simulink model "SCAUN_NOBIL"  (R2020a)
settings: Solver=VariableStepAuto  StartTime=0.0  StopTime=35  RelTol=1e-3
model workspace: external: MATLAB File E:\LICENTA\V6.0 - Model nou rotit Iunie\SCAUN_NOBIL_DataFile1.m (data not in the file)
undefined symbols (not defined in the file or in its folder): magnitude, sigbuilder_block, smiData, X, Y, Z
libraries: sm_lib x88, nesl_utility x19, simulink_extras x1
(part 1 of 3)
settings Model: Creator=Sebastian  LastModifiedBy=Sebastian

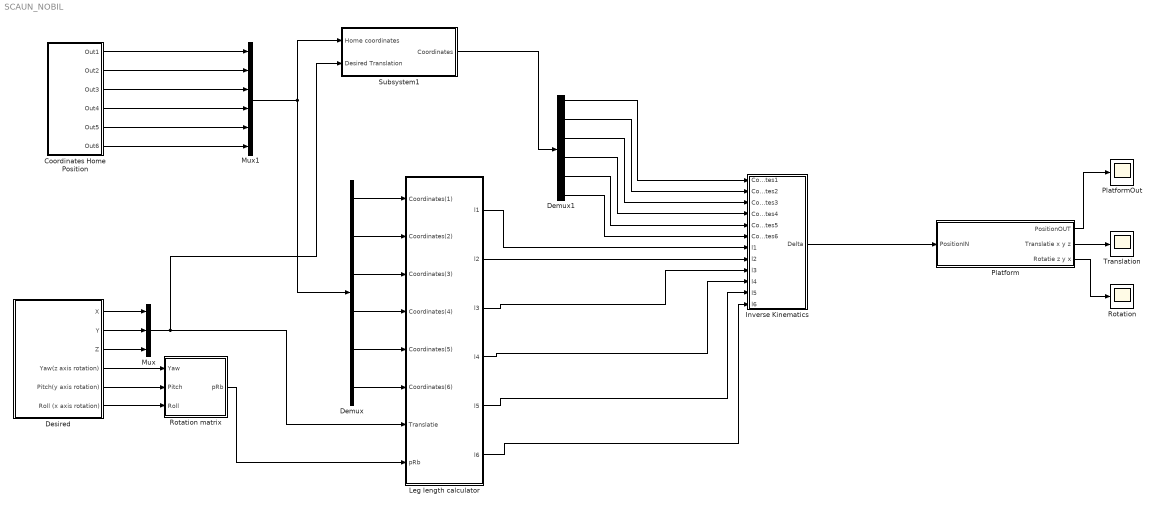
== system SCAUN_NOBIL ==
  Coordinates Home Position : Subsystem  TreatAsAtomicUnit=on
  Demux : Demux  Outputs=6
  Demux1 : Demux  Outputs=6
  Desired : Subsystem
  Inverse Kinematics : Subsystem
  Leg length calculator : Subsystem
  Mux : Mux  Inputs=3
  Mux1 : Mux  Inputs=6
  Platform : Subsystem
  PlatformOut : Scope
  Rotation : Scope
  Rotation matrix : Subsystem
  Subsystem1 : Subsystem
  Translation : Scope
  wires:
  Leg length calculator/6(l6) -> Inverse Kinematics/12(l6)
  Rotation matrix/1(pRb) -> Leg length calculator/8(pRb)
  Desired/2(Y) -> Mux/2
  Subsystem1/1(Coordinates) -> Demux1/1
  Inverse Kinematics/1(Delta) -> Platform/1(PositionIN)
  Platform/1(PositionOUT) -> PlatformOut/1
  Leg length calculator/5(l5) -> Inverse Kinematics/11(l5)
  Leg length calculator/4(l4) -> Inverse Kinematics/10(l4)
  Leg length calculator/3(l3) -> Inverse Kinematics/9(l3)
  Mux1/1 -> Demux/1, Subsystem1/1(Home coordinates)
  Desired/5(Pitch(y axis rotation)) -> Rotation matrix/2(Pitch)
  Coordinates Home Position/3(Out3) -> Mux1/3
  Coordinates Home Position/2(Out2) -> Mux1/2
  Demux1/4 -> Inverse Kinematics/4(Coordinates4)
  Platform/3(Rotatie z y x) -> Rotation/1
  Mux/1 -> Subsystem1/2(Desired Translation), Leg length calculator/7(Translatie)
  Desired/6(Roll (x axis rotation)) -> Rotation matrix/3(Roll)
  Leg length calculator/2(l2) -> Inverse Kinematics/8(l2)
  Coordinates Home Position/5(Out5) -> Mux1/5
  Leg length calculator/1(l1) -> Inverse Kinematics/7(l1)
  Demux/3 -> Leg length calculator/3(Coordinates(3))
  Demux1/5 -> Inverse Kinematics/5(Coordinates5)
  Coordinates Home Position/4(Out4) -> Mux1/4
  Demux/1 -> Leg length calculator/1(Coordinates(1))
  Demux1/1 -> Inverse Kinematics/1(Coordinates1)
  Coordinates Home Position/1(Out1) -> Mux1/1
  Platform/2(Translatie x y z) -> Translation/1
  Demux/5 -> Leg length calculator/5(Coordinates(5))
  Demux/6 -> Leg length calculator/6(Coordinates(6))
  Demux/2 -> Leg length calculator/2(Coordinates(2))
  Demux1/6 -> Inverse Kinematics/6(Coordinates6)
  Desired/1(X) -> Mux/1
  Demux1/2 -> Inverse Kinematics/2(Coordinates2)
  Demux1/3 -> Inverse Kinematics/3(Coordinates3)
  Desired/4(Yaw(z axis rotation)) -> Rotation matrix/1(Yaw)
  Demux/4 -> Leg length calculator/4(Coordinates(4))
  Desired/3(Z) -> Mux/3
  Coordinates Home Position/6(Out6) -> Mux1/6

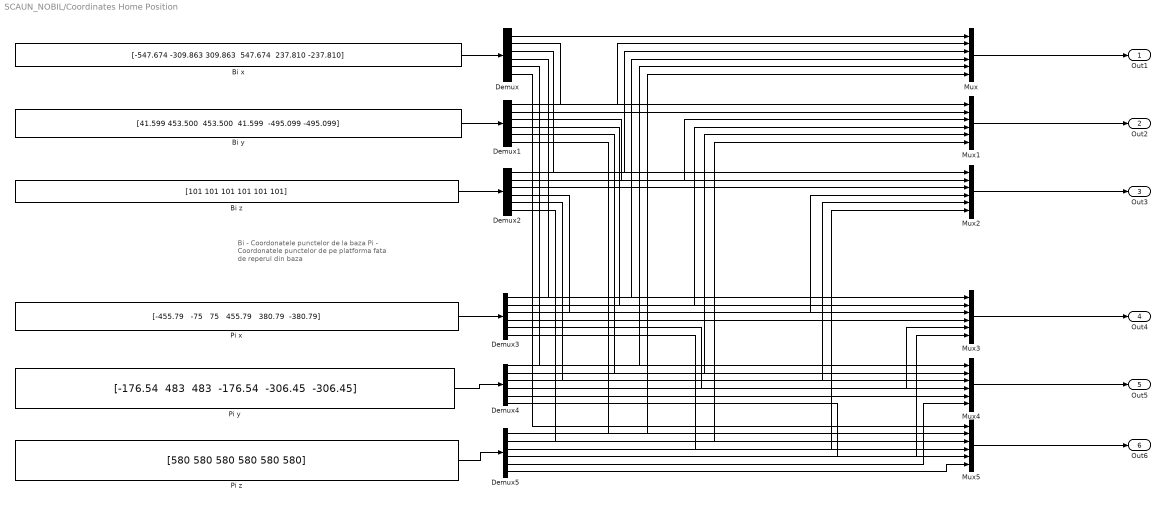
== system SCAUN_NOBIL/Coordinates Home Position ==
  note: Bi - Coordonatele punctelor de la baza
      | Pi - Coordonatele punctelor de pe platforma
      |       fata de reperul din baza
  Bi x : Constant  Value="[-547.674 -309.863 309.863  547.674  237.810 -237.810]"
  Bi y : Constant  Value="[41.599 453.500  453.500  41.599  -495.099 -495.099]"
  Bi z : Constant  Value=[101 101 101 101 101 101]
  Demux{,1..5} (6 alike) : Demux  Outputs=6
  Mux{,1..5} (6 alike) : Mux  Inputs=6
  Pi x : Constant  Value="[-455.79   -75   75   455.79   380.79  -380.79]"
  Pi y : Constant  Value="[-176.54  483  483  -176.54  -306.45  -306.45]"
  Pi z : Constant  Value=[580 580 580 580 580 580]
  Out1 : Outport
  Out2 : Outport  Port=2
  Out3 : Outport  Port=3
  Out4 : Outport  Port=4
  Out5 : Outport  Port=5
  Out6 : Outport  Port=6
  wires:
  Bi x/1 -> Demux/1
  Bi y/1 -> Demux1/1
  Bi z/1 -> Demux2/1
  Pi x/1 -> Demux3/1
  Pi y/1 -> Demux4/1
  Pi z/1 -> Demux5/1
  Demux/1 -> Mux/1
  Demux/2 -> Mux1/1
  Demux/3 -> Mux2/1
  Demux/4 -> Mux3/1
  Demux/5 -> Mux4/1
  Demux/6 -> Mux5/1
  Demux1/1 -> Mux/2
  Demux1/2 -> Mux1/2
  Demux1/3 -> Mux2/2
  Demux1/4 -> Mux3/2
  Demux1/5 -> Mux4/2
  Demux1/6 -> Mux5/2
  Demux2/1 -> Mux/3
  Demux2/2 -> Mux1/3
  Demux2/3 -> Mux2/3
  Demux2/4 -> Mux3/3
  Demux2/5 -> Mux4/3
  Demux2/6 -> Mux5/3
  Demux3/1 -> Mux/4
  Demux3/2 -> Mux1/4
  Demux3/3 -> Mux2/4
  Demux3/4 -> Mux3/4
  Demux3/5 -> Mux4/4
  Demux3/6 -> Mux5/4
  Demux4/1 -> Mux/5
  Demux4/2 -> Mux1/5
  Demux4/3 -> Mux2/5
  Demux4/4 -> Mux3/5
  Demux4/5 -> Mux4/5
  Demux4/6 -> Mux5/5
  Demux5/1 -> Mux/6
  Demux5/2 -> Mux1/6
  Demux5/3 -> Mux2/6
  Demux5/4 -> Mux3/6
  Demux5/5 -> Mux4/6
  Demux5/6 -> Mux5/6
  Mux/1 -> Out1/1
  Mux1/1 -> Out2/1
  Mux2/1 -> Out3/1
  Mux3/1 -> Out4/1
  Mux4/1 -> Out5/1
  Mux5/1 -> Out6/1

== system SCAUN_NOBIL/Desired ==
  MAX_IN : Subsystem  Tag=STV Subsys  LoadFcn=sigbuilder_block('load');  StartFcn=sigbuilder_block('start');  StopFcn=sigbuilder_block('stop');  ClipboardFcn=sigbuilder_block('clipboard');  mask(Sigbuilder block){tuvar=[0:10]}
      mask help: Simulink:masks:SigbuilderBlock_MD
      mask init:
      | if ~strcmp(get_param(bdroot(gcbh),'SimulationStatus'),'stopped') tuvar = sigbuilder_block('maskInit'); end
      settings: CopyFcn=sigbuilder_block('copy');  DeleteFcn=sigbuilder_block('delete');  ModelCloseFcn=sigbuilder_block('modelClose');  PreSaveFcn=sigbuilder_block('preSave');  PauseFcn=sigbuilder_block('pause');  ContinueFcn=sigbuilder_block('continue');  NameChangeFcn=sigbuilder_block('namechange');  OpenFcn=sigbuilder_block('open',[0.75 30.75 718.5 715.5 ]);  CloseFcn=sigbuilder_block('close');
      mask Display: plot(0, 0, 100, 100,[2, 2, 32, 32, 2], [68, 8, 8, 68, 68],[32, 2], [38, 38], [32, 19, 2],[53, 60, 44], [32, 17, 17, 2],[16, 16, 31, 31]);txt = getActiveGroup(gcbh);text(2, 100, txt,'verticalAlignment', 'top');
  X : Outport
  Y : Outport  Port=2
  Z : Outport  Port=3
  Yaw(z axis rotation) : Outport  Port=4
  Pitch(y axis rotation) : Outport  Port=5
  Roll (x axis rotation) : Outport  Port=6
  wires:
  MAX_IN/1(Signal X) -> X/1
  MAX_IN/3(Signal Z) -> Z/1
  MAX_IN/5(Signal Pitch) -> Pitch(y axis rotation)/1
  MAX_IN/6(Signal Roll) -> Roll (x axis rotation)/1
  MAX_IN/2(Signal Y) -> Y/1
  MAX_IN/4(Signal Yaw) -> Yaw(z axis rotation)/1

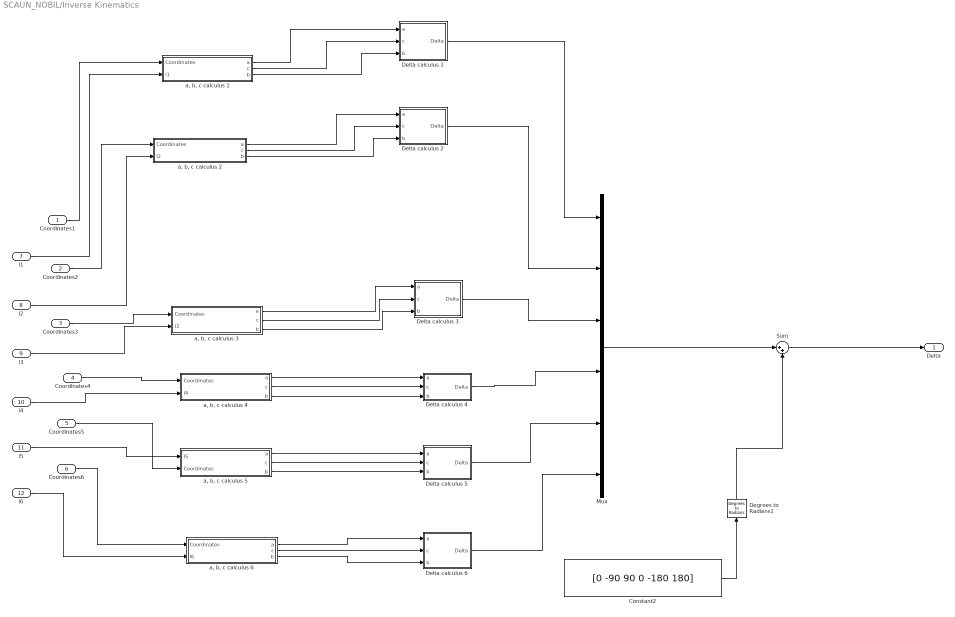
== system SCAUN_NOBIL/Inverse Kinematics ==
  Coordinates1 : Inport
  Coordinates2 : Inport  Port=2
  Coordinates3 : Inport  Port=3
  Coordinates4 : Inport  Port=4
  Coordinates5 : Inport  Port=5
  Coordinates6 : Inport  Port=6
  l1 : Inport  Port=7
  l2 : Inport  Port=8
  l3 : Inport  Port=9
  l4 : Inport  Port=10
  l5 : Inport  Port=11
  l6 : Inport  Port=12
  Constant2 : Constant  Value=[0 -90 90 0 -180 180]
  Degrees to Radians1 : simulink_extras/Transformations/Degrees to Radians
  Delta calculus 1 : Subsystem
  Delta calculus 2 : Subsystem
  Delta calculus 3 : Subsystem
  Delta calculus 4 : Subsystem
  Delta calculus 5 : Subsystem
  Delta calculus 6 : Subsystem
  Mux : Mux  Inputs=6
  Sum : Sum  Inputs=|++
  "a, b, c calculus 1" : Subsystem
  "a, b, c calculus 2" : Subsystem
  "a, b, c calculus 3" : Subsystem
  "a, b, c calculus 4" : Subsystem
  "a, b, c calculus 5" : Subsystem
  "a, b, c calculus 6" : Subsystem
  Delta : Outport
  wires:
  "a, b, c calculus 1"/2(c) -> Delta calculus 1/2(c)
  "a, b, c calculus 1"/1(a) -> Delta calculus 1/1(a)
  "a, b, c calculus 1"/3(b) -> Delta calculus 1/3(b)
  Delta calculus 1/1(Delta) -> Mux/1
  Delta calculus 2/1(Delta) -> Mux/2
  Delta calculus 5/1(Delta) -> Mux/5
  Delta calculus 6/1(Delta) -> Mux/6
  Delta calculus 4/1(Delta) -> Mux/4
  Delta calculus 3/1(Delta) -> Mux/3
  Mux/1 -> Sum/1
  l1/1 -> "a, b, c calculus 1"/2(l1)
  l2/1 -> "a, b, c calculus 2"/2(l2)
  l3/1 -> "a, b, c calculus 3"/2(l3)
  l4/1 -> "a, b, c calculus 4"/2(l4)
  l5/1 -> "a, b, c calculus 5"/1(l5)
  l6/1 -> "a, b, c calculus 6"/2(l6)
  "a, b, c calculus 2"/1(a) -> Delta calculus 2/1(a)
  "a, b, c calculus 2"/2(c) -> Delta calculus 2/2(c)
  "a, b, c calculus 2"/3(b) -> Delta calculus 2/3(b)
  "a, b, c calculus 3"/1(a) -> Delta calculus 3/1(a)
  "a, b, c calculus 3"/2(c) -> Delta calculus 3/2(c)
  "a, b, c calculus 3"/3(b) -> Delta calculus 3/3(b)
  "a, b, c calculus 4"/1(a) -> Delta calculus 4/1(a)
  "a, b, c calculus 4"/2(c) -> Delta calculus 4/2(c)
  "a, b, c calculus 4"/3(b) -> Delta calculus 4/3(b)
  "a, b, c calculus 5"/1(a) -> Delta calculus 5/1(a)
  "a, b, c calculus 5"/2(c) -> Delta calculus 5/2(c)
  "a, b, c calculus 5"/3(b) -> Delta calculus 5/3(b)
  "a, b, c calculus 6"/1(a) -> Delta calculus 6/1(a)
  "a, b, c calculus 6"/2(c) -> Delta calculus 6/2(c)
  "a, b, c calculus 6"/3(b) -> Delta calculus 6/3(b)
  Coordinates1/1 -> "a, b, c calculus 1"/1(Coordinates)
  Coordinates2/1 -> "a, b, c calculus 2"/1(Coordinates)
  Coordinates3/1 -> "a, b, c calculus 3"/1(Coordinates)
  Coordinates4/1 -> "a, b, c calculus 4"/1(Coordinates)
  Coordinates5/1 -> "a, b, c calculus 5"/2(Coordinates)
  Coordinates6/1 -> "a, b, c calculus 6"/1(Coordinates)
  Sum/1 -> Delta/1
  Degrees to Radians1/1 -> Sum/2
  Constant2/1 -> Degrees to Radians1/1

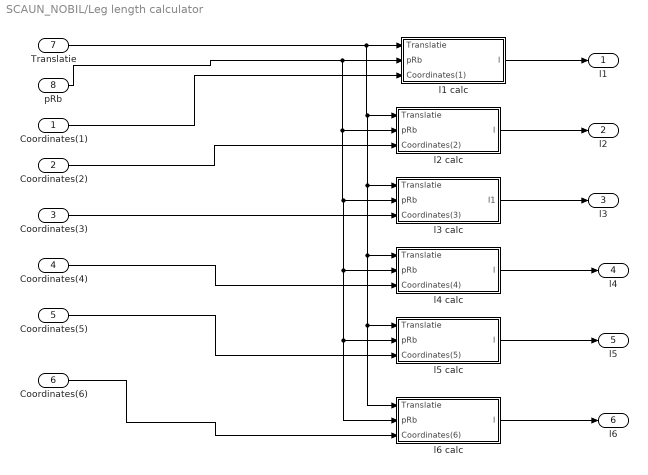
== system SCAUN_NOBIL/Leg length calculator ==
  Coordinates(1) : Inport
  Coordinates(2) : Inport  Port=2
  Coordinates(3) : Inport  Port=3
  Coordinates(4) : Inport  Port=4
  Coordinates(5) : Inport  Port=5
  Coordinates(6) : Inport  Port=6
  Translatie : Inport  Port=7
  pRb : Inport  Port=8
  l1 calc : Subsystem
  l2 calc : Subsystem
  l3 calc : Subsystem
  l4 calc : Subsystem
  l5 calc : Subsystem
  l6 calc : Subsystem
  l1 : Outport
  l2 : Outport  Port=2
  l3 : Outport  Port=3
  l4 : Outport  Port=4
  l5 : Outport  Port=5
  l6 : Outport  Port=6
  wires:
  Coordinates(3)/1 -> l3 calc/3(Coordinates(3))
  Coordinates(6)/1 -> l6 calc/3(Coordinates(6))
  l1 calc/1(l) -> l1/1
  Coordinates(1)/1 -> l1 calc/3(Coordinates(1))
  pRb/1 -> l6 calc/2(pRb), l5 calc/2(pRb), l4 calc/2(pRb), l3 calc/2(pRb), l2 calc/2(pRb), l1 calc/2(pRb)
  Translatie/1 -> l6 calc/1(Translatie), l5 calc/1(Translatie), l4 calc/1(Translatie), l3 calc/1(Translatie), l2 calc/1(Translatie), l1 calc/1(Translatie)
  Coordinates(2)/1 -> l2 calc/3(Coordinates(2))
  l2 calc/1(l) -> l2/1
  Coordinates(5)/1 -> l5 calc/3(Coordinates(5))
  l5 calc/1(l) -> l5/1
  l6 calc/1(l) -> l6/1
  l4 calc/1(l) -> l4/1
  Coordinates(4)/1 -> l4 calc/3(Coordinates(4))
  l3 calc/1(l1) -> l3/1

== system SCAUN_NOBIL/Platform ==
  PositionIN : Inport
  Demux : Demux  Outputs=6
  Mux1 : Mux  Inputs=6
  Stewart Platform : Subsystem
  PositionOUT : Outport
  Translatie x y z : Outport  Port=2
  Rotatie z y x : Outport  Port=3
  wires:
  Stewart Platform/8(Rotatie z y x) -> Rotatie z y x/1
  Stewart Platform/6(Out5) -> Mux1/6
  Stewart Platform/5(Out4) -> Mux1/5
  Stewart Platform/3(Out2) -> Mux1/3
  Stewart Platform/7(Translatie x y z) -> Translatie x y z/1
  Demux/4 -> Stewart Platform/4(Inport)
  Demux/6 -> Stewart Platform/6(Inport2)
  PositionIN/1 -> Demux/1
  Demux/5 -> Stewart Platform/5(Inport1)
  Demux/3 -> Stewart Platform/3(Inport5)
  Stewart Platform/4(Out3) -> Mux1/4
  Mux1/1 -> PositionOUT/1
  Stewart Platform/2(Out1) -> Mux1/2
  Stewart Platform/1(Out6) -> Mux1/1
  Demux/1 -> Stewart Platform/1(Inport3)
  Demux/2 -> Stewart Platform/2(Inport4)

== system SCAUN_NOBIL/Rotation matrix ==
  Yaw : Inport
  Pitch : Inport  Port=2
  Roll : Inport  Port=3
  MATLAB Function : MATLAB Function  TreatAsAtomicUnit=on
  pRb : Outport
  wires:
  Yaw/1 -> MATLAB Function/1(yaw)
  Pitch/1 -> MATLAB Function/2(pitch)
  Roll/1 -> MATLAB Function/3(roll)
  MATLAB Function/1(y) -> pRb/1

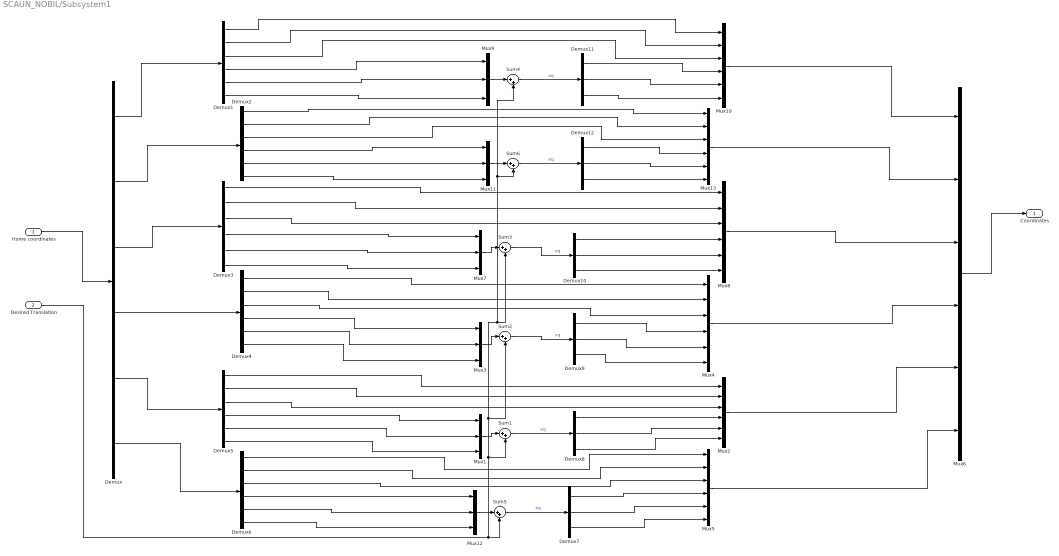
== system SCAUN_NOBIL/Subsystem1 ==
  Home coordinates : Inport
  Desired Translation : Inport  Port=2
  Demux{,1..6} (7 alike) : Demux  Outputs=6
  Demux{7..12} (6 alike) : Demux  Outputs=3
  Mux{1,3,7,9,11..12} (6 alike) : Mux  Inputs=3
  Mux{2,4..6,8,10,13} (7 alike) : Mux  Inputs=6
  Sum{1..6} (6 alike) : Sum  Inputs=|++
  Coordinates : Outport
  wires:
  Home coordinates/1 -> Demux/1
  Demux/1 -> Demux1/1
  Demux/2 -> Demux2/1
  Demux/3 -> Demux3/1
  Demux/4 -> Demux4/1
  Demux/5 -> Demux5/1
  Demux/6 -> Demux6/1
  Demux6/2 -> Mux5/2
  Demux6/3 -> Mux5/3
  Demux6/1 -> Mux5/1
  Sum5/1 -> Demux7/1  "xq"
  Demux6/4 -> Mux12/1
  Demux7/2 -> Mux5/5
  Demux7/1 -> Mux5/4
  Demux6/6 -> Mux12/3
  Mux12/1 -> Sum5/1
  Demux6/5 -> Mux12/2
  Demux7/3 -> Mux5/6
  Mux6/1 -> Coordinates/1
  Mux5/1 -> Mux6/6
  Demux8/1 -> Mux2/4
  Sum1/1 -> Demux8/1  "xq"
  Mux1/1 -> Sum1/1
  Demux8/2 -> Mux2/5
  Demux8/3 -> Mux2/6
  Mux2/1 -> Mux6/5
  Demux5/1 -> Mux2/1
  Demux5/2 -> Mux2/2
  Demux5/3 -> Mux2/3
  Demux5/4 -> Mux1/1
  Demux5/5 -> Mux1/2
  Demux5/6 -> Mux1/3
  Demux9/3 -> Mux4/6
  Demux9/2 -> Mux4/5
  Mux3/1 -> Sum2/1
  Demux4/5 -> Mux3/2
  Demux9/1 -> Mux4/4
  Demux4/6 -> Mux3/3
  Demux4/1 -> Mux4/1
  Demux4/2 -> Mux4/2
  Demux4/3 -> Mux4/3
  Demux4/4 -> Mux3/1
  Sum2/1 -> Demux9/1  "xq"
  Mux4/1 -> Mux6/4
  Demux10/3 -> Mux8/6
  Demux10/2 -> Mux8/5
  Mux7/1 -> Sum3/1
  Demux3/5 -> Mux7/2
  Demux10/1 -> Mux8/4
  Demux3/6 -> Mux7/3
  Demux3/1 -> Mux8/1
  Demux3/2 -> Mux8/2
  Demux3/3 -> Mux8/3
  Demux3/4 -> Mux7/1
  Sum3/1 -> Demux10/1  "xq"
  Mux8/1 -> Mux6/3
  Demux12/3 -> Mux13/6
  Demux12/2 -> Mux13/5
  Mux11/1 -> Sum6/1
  Demux2/5 -> Mux11/2
  Demux12/1 -> Mux13/4
  Demux2/6 -> Mux11/3
  Demux2/1 -> Mux13/1
  Demux2/2 -> Mux13/2
  Demux2/3 -> Mux13/3
  Demux2/4 -> Mux11/1
  Sum6/1 -> Demux12/1  "xq"
  Mux13/1 -> Mux6/2
  Demux11/3 -> Mux10/6
  Demux11/2 -> Mux10/5
  Mux9/1 -> Sum4/1
  Demux1/5 -> Mux9/2
  Demux11/1 -> Mux10/4
  Demux1/6 -> Mux9/3
  Demux1/1 -> Mux10/1
  Demux1/2 -> Mux10/2
  Demux1/3 -> Mux10/3
  Demux1/4 -> Mux9/1
  Sum4/1 -> Demux11/1  "xq"
  Mux10/1 -> Mux6/1
  Desired Translation/1 -> Sum5/2, Sum3/2, Sum4/2, Sum6/2, Sum2/2, Sum1/2

== system SCAUN_NOBIL/Desired/MAX_IN ==
  Demux : Demux  Tag=STV Demux  Outputs=6
      settings: DisplayOption=none
  FromWs : FromWorkspace  Tag=STV FromWs  VariableName=tuvar
      SigBuilderData=|
      | common.afterFinalStr = 'Extrapolate'
      | common.sampleTime = 0
      | dataSet.timeRange = [0 35]
      | dataSet.name = 'Group 1'
      | sbobj.Groups.Name = 'Group 1'
      | sbobj.Groups.Signals(1).Name = 'Signal X'
      | sbobj.Groups.Signals(1).XData = [0 1.5 3 5 5.46 35]
      | sbobj.Groups.Signals(1).YData = [1 0 150 -150 0 0]
      | sbobj.Groups.Signals(2).Name = 'Signal Y'
      | sbobj.Groups.Signals(2).XData = [0 6.5 8 10 10.5 35]
      | sbobj.Groups.Signals(2).YData = [5 5 150 -155 0 5]
      | sbobj.Groups.Signals(3).Name = 'Signal Z'
      | sbobj.Groups.Signals(3).XData = [0 11 13.5 16 16.62 35]
      | sbobj.Groups.Signals(3).YData = [-1 -1 100 -120 0 -1]
      | sbobj.Groups.Signals(4).Name = 'Signal Yaw'
      | sbobj.Groups.Signals(4).XData = [0 17 19.5 22 22.68 35]
      | sbobj.Groups.Signals(4).YData = [0 0 0.3 -0.3 0 0]
      | sbobj.Groups.Signals(5).Name = 'Signal Pitch'
      | sbobj.Groups.Signals(5).XData = [0 23 25.5 28 28.42 35]
      | sbobj.Groups.Signals(5).YData = [0 0 0.115 -0.12 0 0]
      | sbobj.Groups.Signals(6).Name = 'Signal Roll'
      | sbobj.Groups.Signals(6).XData = [0 30 30 32.5 34.62 35]
      | sbobj.Groups.Signals(6).YData = [0 0 0.002 0.16 -0.16 0]
      | sbobj.Groups.TimeRange = [0 35]
  Signal X : Outport  Tag=STV Outport
  Signal Y : Outport  Tag=STV Outport  Port=2
  Signal Z : Outport  Tag=STV Outport  Port=3
  Signal Yaw : Outport  Tag=STV Outport  Port=4
  Signal Pitch : Outport  Tag=STV Outport  Port=5
  Signal Roll : Outport  Tag=STV Outport  Port=6
  wires:
  FromWs/1 -> Demux/1
  Demux/1 -> Signal X/1
  Demux/2 -> Signal Y/1
  Demux/3 -> Signal Z/1
  Demux/4 -> Signal Yaw/1
  Demux/5 -> Signal Pitch/1
  Demux/6 -> Signal Roll/1

== system SCAUN_NOBIL/Inverse Kinematics/Delta calculus 1 ==
  a : Inport
  c : Inport  Port=2
  b : Inport  Port=3
  Asin5 : Trigonometry  Operator=asin
  Atan6 : Trigonometry  Operator=atan
  Divide10 : Product  Inputs=*/
  Divide11 : Product  Inputs=*/
  Math Function11 : Math  Operator=magnitude^2  SaturateOnIntegerOverflow=on
  Math Function12 : Math  Operator=magnitude^2  SaturateOnIntegerOverflow=on
  Square Root5 : Sqrt  SaturateOnIntegerOverflow=on
  Sum11 : Sum  Inputs=++|
  Sum12 : Sum  Inputs=|+-
  Delta : Outport
  wires:
  Math Function11/1 -> Sum11/1
  Math Function12/1 -> Sum11/2
  Divide11/1 -> Atan6/1
  Asin5/1 -> Sum12/1
  Sum11/1 -> Square Root5/1
  Divide10/1 -> Asin5/1
  Atan6/1 -> Sum12/2
  b/1 -> Math Function12/1, Divide11/1
  a/1 -> Divide11/2, Math Function11/1
  Sum12/1 -> Delta/1
  Square Root5/1 -> Divide10/2
  c/1 -> Divide10/1

== system SCAUN_NOBIL/Inverse Kinematics/Delta calculus 2 ==
  a : Inport
  c : Inport  Port=2
  b : Inport  Port=3
  Asin5 : Trigonometry  Operator=asin  OutputSignalType=real
  Atan6 : Trigonometry  Operator=atan
  Display11 : Display
  Divide10 : Product  Inputs=*/
  Divide11 : Product  Inputs=*/
  Math Function11 : Math  Operator=magnitude^2  SaturateOnIntegerOverflow=on
  Math Function12 : Math  Operator=magnitude^2  SaturateOnIntegerOverflow=on
  Square Root5 : Sqrt  SaturateOnIntegerOverflow=on
  Sum11 : Sum  Inputs=++|
  Sum12 : Sum  Inputs=|+-
  Delta : Outport
  wires:
  Math Function11/1 -> Sum11/1
  Math Function12/1 -> Sum11/2
  a/1 -> Divide11/2, Math Function11/1
  Asin5/1 -> Sum12/1
  b/1 -> Math Function12/1, Divide11/1
  Divide10/1 -> Asin5/1
  Atan6/1 -> Sum12/2
  Divide11/1 -> Atan6/1
  c/1 -> Divide10/1
  Sum11/1 -> Square Root5/1
  Sum12/1 -> Delta/1
  Square Root5/1 -> Display11/1, Divide10/2

== system SCAUN_NOBIL/Inverse Kinematics/Delta calculus 3 ==
  a : Inport
  c : Inport  Port=2
  b : Inport  Port=3
  Asin5 : Trigonometry  Operator=asin  OutputSignalType=real
  Atan6 : Trigonometry  Operator=atan
  Divide10 : Product  Inputs=*/
  Divide11 : Product  Inputs=*/
  Math Function11 : Math  Operator=magnitude^2  SaturateOnIntegerOverflow=on
  Math Function12 : Math  Operator=magnitude^2  SaturateOnIntegerOverflow=on
  Square Root5 : Sqrt  SaturateOnIntegerOverflow=on
  Sum11 : Sum  Inputs=++|
  Sum12 : Sum  Inputs=|+-
  Delta : Outport
  wires:
  Math Function11/1 -> Sum11/1
  Math Function12/1 -> Sum11/2
  a/1 -> Divide11/2, Math Function11/1
  Asin5/1 -> Sum12/1
  b/1 -> Math Function12/1, Divide11/1
  Divide10/1 -> Asin5/1
  Atan6/1 -> Sum12/2
  Divide11/1 -> Atan6/1
  Sum11/1 -> Square Root5/1
  Square Root5/1 -> Divide10/2
  Sum12/1 -> Delta/1
  c/1 -> Divide10/1

== system SCAUN_NOBIL/Inverse Kinematics/Delta calculus 4 ==
  a : Inport
  c : Inport  Port=2
  b : Inport  Port=3
  Asin5 : Trigonometry  Operator=asin  OutputSignalType=real
  Atan6 : Trigonometry  Operator=atan
  Divide10 : Product  Inputs=*/
  Divide11 : Product  Inputs=*/
  Math Function11 : Math  Operator=magnitude^2  SaturateOnIntegerOverflow=on
  Math Function12 : Math  Operator=magnitude^2  SaturateOnIntegerOverflow=on
  Square Root5 : Sqrt  SaturateOnIntegerOverflow=on
  Sum11 : Sum  Inputs=++|
  Sum12 : Sum  Inputs=|+-
  Delta : Outport
  wires:
  Math Function11/1 -> Sum11/1
  Math Function12/1 -> Sum11/2
  a/1 -> Divide11/2, Math Function11/1
  Asin5/1 -> Sum12/1
  b/1 -> Math Function12/1, Divide11/1
  Divide10/1 -> Asin5/1
  Atan6/1 -> Sum12/2
  Divide11/1 -> Atan6/1
  c/1 -> Divide10/1
  Sum11/1 -> Square Root5/1
  Square Root5/1 -> Divide10/2
  Sum12/1 -> Delta/1

== system SCAUN_NOBIL/Inverse Kinematics/Delta calculus 5 ==
  a : Inport
  c : Inport  Port=2
  b : Inport  Port=3
  Asin5 : Trigonometry  Operator=asin  OutputSignalType=real
  Atan6 : Trigonometry  Operator=atan
  Divide10 : Product  Inputs=*/
  Divide11 : Product  Inputs=*/
  Math Function11 : Math  Operator=magnitude^2  SaturateOnIntegerOverflow=on
  Math Function12 : Math  Operator=magnitude^2  SaturateOnIntegerOverflow=on
  Square Root5 : Sqrt  SaturateOnIntegerOverflow=on
  Sum11 : Sum  Inputs=++|
  Sum12 : Sum  Inputs=|+-
  Delta : Outport
  wires:
  Math Function11/1 -> Sum11/1
  Math Function12/1 -> Sum11/2
  a/1 -> Divide11/2, Math Function11/1
  Asin5/1 -> Sum12/1
  b/1 -> Math Function12/1, Divide11/1
  Divide10/1 -> Asin5/1
  Atan6/1 -> Sum12/2
  Divide11/1 -> Atan6/1
  Sum11/1 -> Square Root5/1
  Sum12/1 -> Delta/1
  Square Root5/1 -> Divide10/2
  c/1 -> Divide10/1

== system SCAUN_NOBIL/Inverse Kinematics/Delta calculus 6 ==
  a : Inport
  c : Inport  Port=2
  b : Inport  Port=3
  Asin5 : Trigonometry  Operator=asin  OutputSignalType=real
  Atan6 : Trigonometry  Operator=atan
  Divide10 : Product  Inputs=*/
  Divide11 : Product  Inputs=*/
  Math Function11 : Math  Operator=magnitude^2  SaturateOnIntegerOverflow=on
  Math Function12 : Math  Operator=magnitude^2  SaturateOnIntegerOverflow=on
  Square Root5 : Sqrt  SaturateOnIntegerOverflow=on
  Sum11 : Sum  Inputs=++|
  Sum12 : Sum  Inputs=|+-
  Delta : Outport
  wires:
  Math Function11/1 -> Sum11/1
  Sum12/1 -> Delta/1
  Math Function12/1 -> Sum11/2
  a/1 -> Divide11/2, Math Function11/1
  Asin5/1 -> Sum12/1
  b/1 -> Math Function12/1, Divide11/1
  Divide10/1 -> Asin5/1
  Atan6/1 -> Sum12/2
  Divide11/1 -> Atan6/1
  c/1 -> Divide10/1
  Sum11/1 -> Square Root5/1
  Square Root5/1 -> Divide10/2

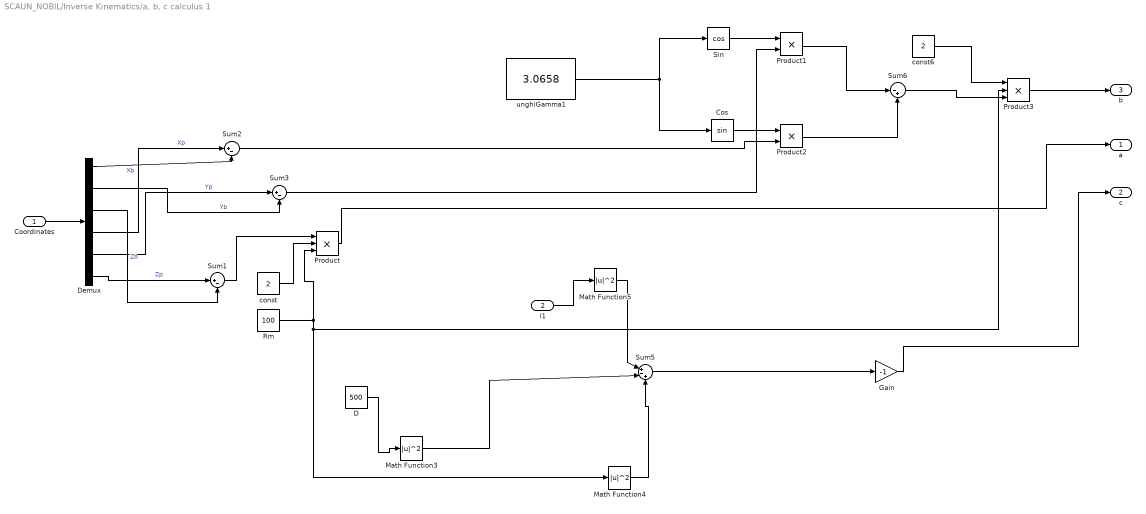
== system SCAUN_NOBIL/Inverse Kinematics/a, b, c calculus 1 ==
  Coordinates : Inport
  l1 : Inport  Port=2
  Cos : Trigonometry
  D : Constant  Value=500
  Demux : Demux  Outputs=6
  Gain : Gain  Gain=-1
  Math Function3 : Math  Operator=magnitude^2  SaturateOnIntegerOverflow=on
  Math Function4 : Math  Operator=magnitude^2  SaturateOnIntegerOverflow=on
  Math Function5 : Math  Operator=magnitude^2  SaturateOnIntegerOverflow=on
  Product : Product  Inputs=3
  Product1 : Product
  Product2 : Product
  Product3 : Product  Inputs=3
  Rm : Constant  Value=100
  Sin : Trigonometry  Operator=cos
  Sum1 : Sum  Inputs=|+-
  Sum2 : Sum  Inputs=|+-
  Sum3 : Sum  Inputs=|+-
  Sum5 : Sum  Inputs=|+-+
  Sum6 : Sum  Inputs=|-+
  const : Constant  Value=2
  const6 : Constant  Value=2
  unghiGamma1 : Constant  Value=3.0658
  a : Outport
  c : Outport  Port=2
  b : Outport  Port=3
  wires:
  Demux/2 -> Sum3/2  "Yb"
  Demux/4 -> Sum2/1  "Xp"
  Demux/5 -> Sum3/1  "Yp"
  Demux/1 -> Sum2/2  "Xb"
  unghiGamma1/1 -> Sin/1, Cos/1
  Math Function4/1 -> Sum5/3
  Product/1 -> a/1
  Sin/1 -> Product1/1
  const6/1 -> Product3/1
  Product2/1 -> Sum6/2
  Demux/3 -> Sum1/2  "Zb"
  Product1/1 -> Sum6/1
  Demux/6 -> Sum1/1  "Zp"
  Product3/1 -> b/1
  Sum6/1 -> Product3/3
  Cos/1 -> Product2/1
  Math Function3/1 -> Sum5/2
  Rm/1 -> Math Function4/1, Product3/2, Product/3
  Sum1/1 -> Product/1
  const/1 -> Product/2
  D/1 -> Math Function3/1
  Coordinates/1 -> Demux/1
  l1/1 -> Math Function5/1
  Math Function5/1 -> Sum5/1
  Sum5/1 -> Gain/1
  Gain/1 -> c/1
  Sum3/1 -> Product1/2
  Sum2/1 -> Product2/2

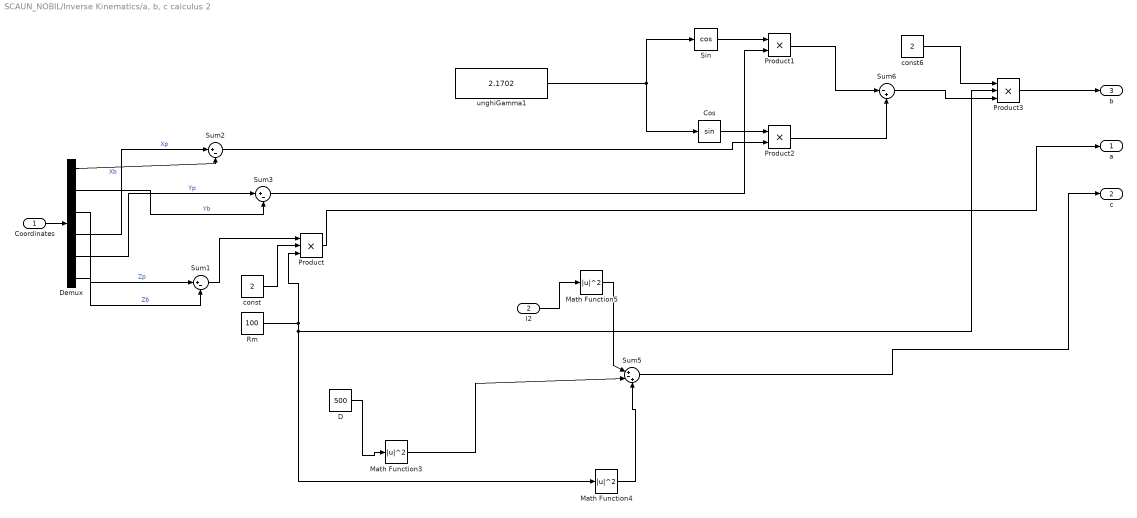
== system SCAUN_NOBIL/Inverse Kinematics/a, b, c calculus 2 ==
  Coordinates : Inport
  l2 : Inport  Port=2
  Cos : Trigonometry
  D : Constant  Value=500
  Demux : Demux  Outputs=6
  Math Function3 : Math  Operator=magnitude^2  SaturateOnIntegerOverflow=on
  Math Function4 : Math  Operator=magnitude^2  SaturateOnIntegerOverflow=on
  Math Function5 : Math  Operator=magnitude^2  SaturateOnIntegerOverflow=on
  Product : Product  Inputs=3
  Product1 : Product
  Product2 : Product
  Product3 : Product  Inputs=3
  Rm : Constant  Value=100
  Sin : Trigonometry  Operator=cos
  Sum1 : Sum  Inputs=|+-
  Sum2 : Sum  Inputs=|+-
  Sum3 : Sum  Inputs=|+-
  Sum5 : Sum  Inputs=|+-+
  Sum6 : Sum  Inputs=|-+
  const : Constant  Value=2
  const6 : Constant  Value=2
  unghiGamma1 : Constant  Value=2.1702
  a : Outport
  c : Outport  Port=2
  b : Outport  Port=3
  wires:
  Math Function5/1 -> Sum5/1
  Product1/1 -> Sum6/1
  Demux/2 -> Sum3/2  "Yb"
  Sum5/1 -> c/1
  Sin/1 -> Product1/1
  Product2/1 -> Sum6/2
  Rm/1 -> Math Function4/1, Product3/2, Product/3
  unghiGamma1/1 -> Sin/1, Cos/1
  Demux/1 -> Sum2/2  "Xb"
  Demux/5 -> Sum3/1  "Yp"
  Demux/4 -> Sum2/1  "Xp"
  const6/1 -> Product3/1
  Coordinates/1 -> Demux/1
  Math Function4/1 -> Sum5/3
  Demux/6 -> Sum1/1  "Zp"
  Demux/3 -> Sum1/2  "Zb"
  D/1 -> Math Function3/1
  Sum6/1 -> Product3/3
  Sum1/1 -> Product/1
  Product3/1 -> b/1
  const/1 -> Product/2
  Math Function3/1 -> Sum5/2
  Product/1 -> a/1
  l2/1 -> Math Function5/1
  Cos/1 -> Product2/1
  Sum3/1 -> Product1/2
  Sum2/1 -> Product2/2

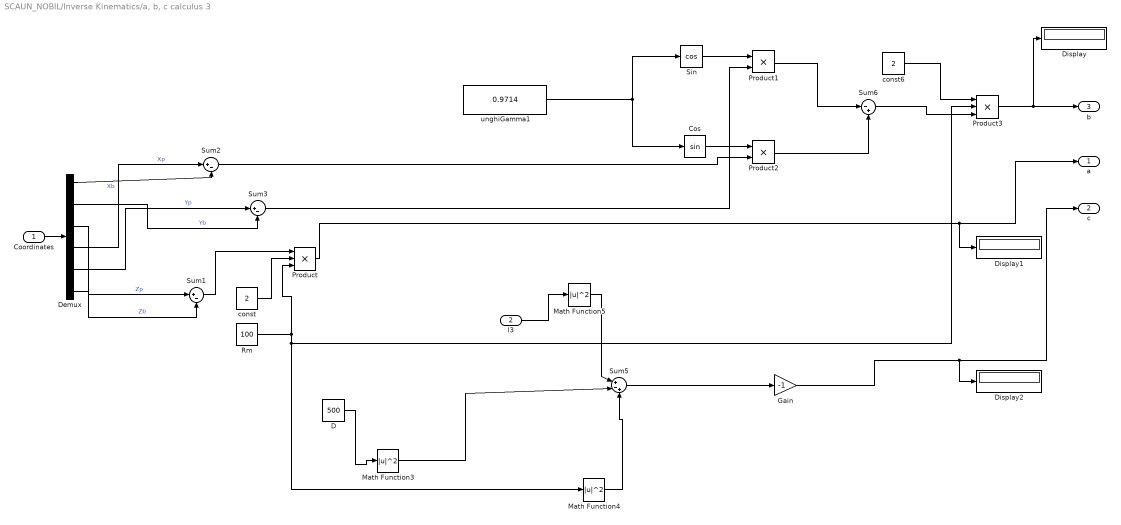
== system SCAUN_NOBIL/Inverse Kinematics/a, b, c calculus 3 ==
  Coordinates : Inport
  l3 : Inport  Port=2
  Cos : Trigonometry
  D : Constant  Value=500
  Demux : Demux  Outputs=6
  Display : Display
  Display1 : Display
  Display2 : Display
  Gain : Gain  Gain=-1
  Math Function3 : Math  Operator=magnitude^2  SaturateOnIntegerOverflow=on
  Math Function4 : Math  Operator=magnitude^2  SaturateOnIntegerOverflow=on
  Math Function5 : Math  Operator=magnitude^2  SaturateOnIntegerOverflow=on
  Product : Product  Inputs=3
  Product1 : Product
  Product2 : Product
  Product3 : Product  Inputs=3
  Rm : Constant  Value=100
  Sin : Trigonometry  Operator=cos
  Sum1 : Sum  Inputs=|+-
  Sum2 : Sum  Inputs=|+-
  Sum3 : Sum  Inputs=|+-
  Sum5 : Sum  Inputs=|+-+
  Sum6 : Sum  Inputs=|-+
  const : Constant  Value=2
  const6 : Constant  Value=2
  unghiGamma1 : Constant  Value=0.9714
  a : Outport
  c : Outport  Port=2
  b : Outport  Port=3
  wires:
  Math Function5/1 -> Sum5/1
  Product1/1 -> Sum6/1
  Demux/2 -> Sum3/2  "Yb"
  Sin/1 -> Product1/1
  Product2/1 -> Sum6/2
  Rm/1 -> Math Function4/1, Product3/2, Product/3
  unghiGamma1/1 -> Sin/1, Cos/1
  Demux/1 -> Sum2/2  "Xb"
  Demux/5 -> Sum3/1  "Yp"
  Demux/4 -> Sum2/1  "Xp"
  const6/1 -> Product3/1
  Coordinates/1 -> Demux/1
  Math Function4/1 -> Sum5/3
  Demux/6 -> Sum1/1  "Zp"
  Demux/3 -> Sum1/2  "Zb"
  D/1 -> Math Function3/1
  Sum6/1 -> Product3/3
  Sum1/1 -> Product/1
  Product3/1 -> Display/1, b/1
  const/1 -> Product/2
  Math Function3/1 -> Sum5/2
  Product/1 -> Display1/1, a/1
  l3/1 -> Math Function5/1
  Cos/1 -> Product2/1
  Sum5/1 -> Gain/1
  Gain/1 -> Display2/1, c/1
  Sum3/1 -> Product1/2
  Sum2/1 -> Product2/2

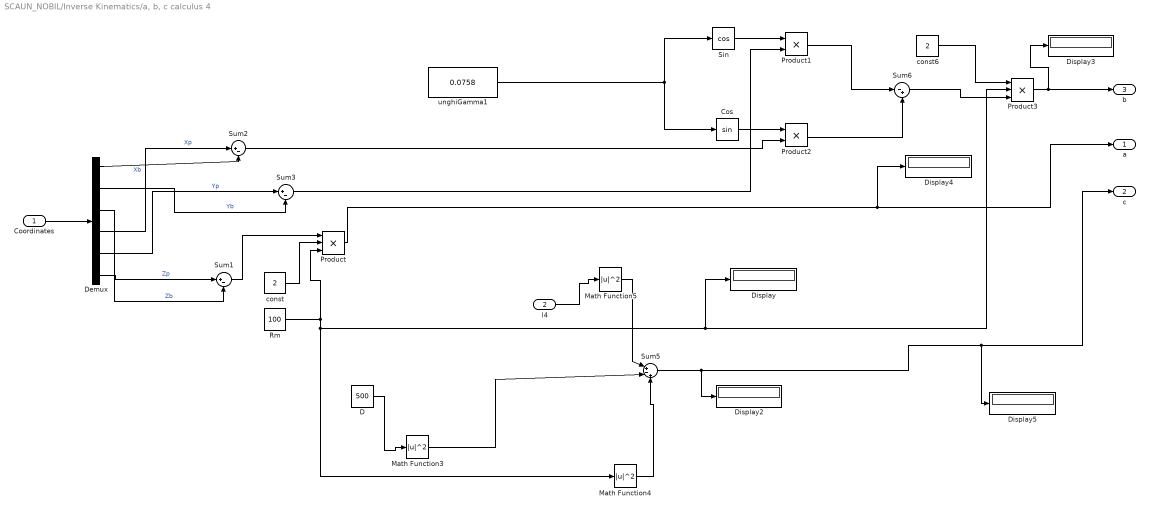
== system SCAUN_NOBIL/Inverse Kinematics/a, b, c calculus 4 ==
  Coordinates : Inport
  l4 : Inport  Port=2
  Cos : Trigonometry
  D : Constant  Value=500
  Demux : Demux  Outputs=6
  Display{,2..5} (5 alike) : Display
  Math Function3 : Math  Operator=magnitude^2  SaturateOnIntegerOverflow=on
  Math Function4 : Math  Operator=magnitude^2  SaturateOnIntegerOverflow=on
  Math Function5 : Math  Operator=magnitude^2  SaturateOnIntegerOverflow=on
  Product : Product  Inputs=3
  Product1 : Product
  Product2 : Product
  Product3 : Product  Inputs=3
  Rm : Constant  Value=100
  Sin : Trigonometry  Operator=cos
  Sum1 : Sum  Inputs=|+-
  Sum2 : Sum  Inputs=|+-
  Sum3 : Sum  Inputs=|+-
  Sum5 : Sum  Inputs=|+-+
  Sum6 : Sum  Inputs=|-+
  const : Constant  Value=2
  const6 : Constant  Value=2
  unghiGamma1 : Constant  Value=0.0758
  a : Outport
  c : Outport  Port=2
  b : Outport  Port=3
  wires:
  Math Function5/1 -> Sum5/1
  Product1/1 -> Sum6/1
  Demux/2 -> Sum3/2  "Yb"
  Sum5/1 -> Display2/1, c/1, Display5/1
  Sin/1 -> Product1/1
  Product2/1 -> Sum6/2
  Rm/1 -> Math Function4/1, Display/1, Product3/2, Product/3
  unghiGamma1/1 -> Sin/1, Cos/1
  Demux/1 -> Sum2/2  "Xb"
  Demux/5 -> Sum3/1  "Yp"
  Demux/4 -> Sum2/1  "Xp"
  const6/1 -> Product3/1
  Coordinates/1 -> Demux/1
  Math Function4/1 -> Sum5/3
  Demux/6 -> Sum1/1  "Zp"
  Demux/3 -> Sum1/2  "Zb"
  D/1 -> Math Function3/1
  Sum6/1 -> Product3/3
  Sum1/1 -> Product/1
  Product3/1 -> Display3/1, b/1
  const/1 -> Product/2
  Math Function3/1 -> Sum5/2
  Product/1 -> a/1, Display4/1
  l4/1 -> Math Function5/1
  Cos/1 -> Product2/1
  Sum2/1 -> Product2/2
  Sum3/1 -> Product1/2

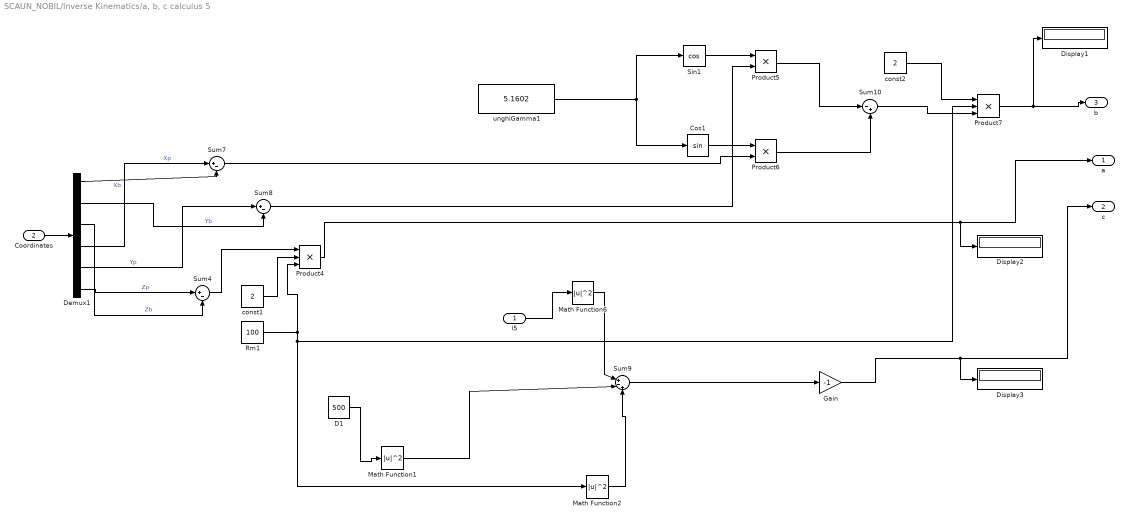
== system SCAUN_NOBIL/Inverse Kinematics/a, b, c calculus 5 ==
  l5 : Inport
  Coordinates : Inport  Port=2
  Cos1 : Trigonometry
  D1 : Constant  Value=500
  Demux1 : Demux  Outputs=6
  Display1 : Display
  Display2 : Display
  Display3 : Display
  Gain : Gain  Gain=-1
  Math Function1 : Math  Operator=magnitude^2  SaturateOnIntegerOverflow=on
  Math Function2 : Math  Operator=magnitude^2  SaturateOnIntegerOverflow=on
  Math Function6 : Math  Operator=magnitude^2  SaturateOnIntegerOverflow=on
  Product4 : Product  Inputs=3
  Product5 : Product
  Product6 : Product
  Product7 : Product  Inputs=3
  Rm1 : Constant  Value=100
  Sin1 : Trigonometry  Operator=cos
  Sum10 : Sum  Inputs=|-+
  Sum4 : Sum  Inputs=|+-
  Sum7 : Sum  Inputs=|+-
  Sum8 : Sum  Inputs=|+-
  Sum9 : Sum  Inputs=|+-+
  const1 : Constant  Value=2
  const2 : Constant  Value=2
  unghiGamma1 : Constant  Value=5.1602
  a : Outport
  c : Outport  Port=2
  b : Outport  Port=3
  wires:
  Sum9/1 -> Gain/1
  Cos1/1 -> Product6/1
  Product4/1 -> a/1, Display2/1
  Demux1/5 -> Sum8/1  "Yp"
  Product6/1 -> Sum10/2
  D1/1 -> Math Function1/1
  Rm1/1 -> Math Function2/1, Product7/2, Product4/3
  l5/1 -> Math Function6/1
  Demux1/6 -> Sum4/1  "Zp"
  const2/1 -> Product7/1
  Sum10/1 -> Product7/3
  Demux1/3 -> Sum4/2  "Zb"
  const1/1 -> Product4/2
  Product7/1 -> b/1, Display1/1
  Sum4/1 -> Product4/1
  Coordinates/1 -> Demux1/1
  Demux1/1 -> Sum7/2  "Xb"
  Math Function2/1 -> Sum9/3
  Math Function6/1 -> Sum9/1
  Demux1/4 -> Sum7/1  "Xp"
  unghiGamma1/1 -> Sin1/1, Cos1/1
  Sin1/1 -> Product5/1
  Math Function1/1 -> Sum9/2
  Demux1/2 -> Sum8/2  "Yb"
  Product5/1 -> Sum10/1
  Gain/1 -> c/1, Display3/1
  Sum8/1 -> Product5/2
  Sum7/1 -> Product6/2

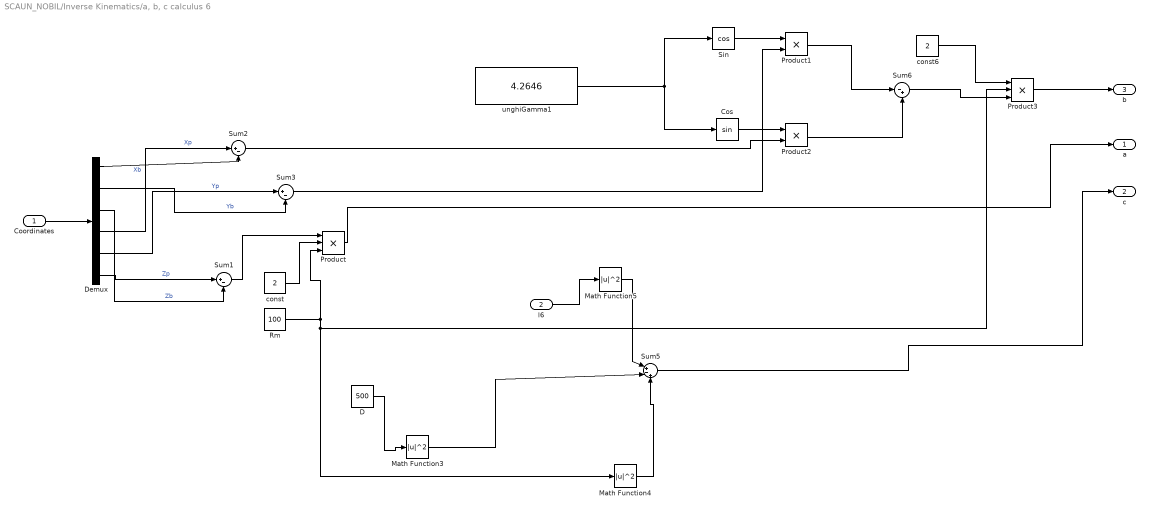
== system SCAUN_NOBIL/Inverse Kinematics/a, b, c calculus 6 ==
  Coordinates : Inport
  l6 : Inport  Port=2
  Cos : Trigonometry
  D : Constant  Value=500
  Demux : Demux  Outputs=6
  Math Function3 : Math  Operator=magnitude^2  SaturateOnIntegerOverflow=on
  Math Function4 : Math  Operator=magnitude^2  SaturateOnIntegerOverflow=on
  Math Function5 : Math  Operator=magnitude^2  SaturateOnIntegerOverflow=on
  Product : Product  Inputs=3
  Product1 : Product
  Product2 : Product
  Product3 : Product  Inputs=3
  Rm : Constant  Value=100
  Sin : Trigonometry  Operator=cos
  Sum1 : Sum  Inputs=|+-
  Sum2 : Sum  Inputs=|+-
  Sum3 : Sum  Inputs=|+-
  Sum5 : Sum  Inputs=|+-+
  Sum6 : Sum  Inputs=|-+
  const : Constant  Value=2
  const6 : Constant  Value=2
  unghiGamma1 : Constant  Value=4.2646
  a : Outport
  c : Outport  Port=2
  b : Outport  Port=3
  wires:
  Math Function5/1 -> Sum5/1
  Product1/1 -> Sum6/1
  Demux/2 -> Sum3/2  "Yb"
  Sum5/1 -> c/1
  Sin/1 -> Product1/1
  Product2/1 -> Sum6/2
  Rm/1 -> Math Function4/1, Product3/2, Product/3
  unghiGamma1/1 -> Sin/1, Cos/1
  Demux/1 -> Sum2/2  "Xb"
  Demux/5 -> Sum3/1  "Yp"
  Demux/4 -> Sum2/1  "Xp"
  const6/1 -> Product3/1
  Coordinates/1 -> Demux/1
  Math Function4/1 -> Sum5/3
  Demux/6 -> Sum1/1  "Zp"
  Demux/3 -> Sum1/2  "Zb"
  D/1 -> Math Function3/1
  Sum6/1 -> Product3/3
  Sum1/1 -> Product/1
  Product3/1 -> b/1
  const/1 -> Product/2
  Math Function3/1 -> Sum5/2
  Product/1 -> a/1
  l6/1 -> Math Function5/1
  Cos/1 -> Product2/1
  Sum3/1 -> Product1/2
  Sum2/1 -> Product2/2

== system SCAUN_NOBIL/Leg length calculator/l1 calc ==
  Translatie : Inport
  pRb : Inport  Port=2
  Coordinates(1) : Inport  Port=3
  Demux : Demux  Outputs=6
  Demux1 : Demux  Outputs=3
  Math Function11 : Math  Operator=magnitude^2  SaturateOnIntegerOverflow=on
  Math Function2 : Math  Operator=magnitude^2  SaturateOnIntegerOverflow=on
  Math Function3 : Math  Operator=magnitude^2  SaturateOnIntegerOverflow=on
  MatrixMultiply : Product  Multiplication=Matrix(*)
  Mux : Mux  Inputs=3
  Mux1 : Mux  Inputs=3
  Sqrt : Sqrt  SaturateOnIntegerOverflow=on
  Sum1 : Sum  Inputs=|++-
  Sum2 : Sum  Inputs=|+++
  l : Outport
  wires:
  Demux/1 -> Mux/1
  Demux/2 -> Mux/2
  Demux/3 -> Mux/3
  Demux/4 -> Mux1/1
  Demux/5 -> Mux1/2
  Demux/6 -> Mux1/3
  Coordinates(1)/1 -> Demux/1
  Mux1/1 -> MatrixMultiply/2  "p1"
  Mux/1 -> Sum1/3  "b1"
  pRb/1 -> MatrixMultiply/1
  MatrixMultiply/1 -> Sum1/2
  Translatie/1 -> Sum1/1
  Demux1/1 -> Math Function11/1
  Math Function11/1 -> Sum2/1
  Math Function2/1 -> Sum2/2
  Demux1/2 -> Math Function2/1
  Demux1/3 -> Math Function3/1
  Sum2/1 -> Sqrt/1
  Sqrt/1 -> l/1
  Sum1/1 -> Demux1/1
  Math Function3/1 -> Sum2/3

== system SCAUN_NOBIL/Leg length calculator/l2 calc ==
  Translatie : Inport
  pRb : Inport  Port=2
  Coordinates(2) : Inport  Port=3
  Demux : Demux  Outputs=6
  Demux1 : Demux  Outputs=3
  Math Function11 : Math  Operator=magnitude^2  SaturateOnIntegerOverflow=on
  Math Function2 : Math  Operator=magnitude^2  SaturateOnIntegerOverflow=on
  Math Function3 : Math  Operator=magnitude^2  SaturateOnIntegerOverflow=on
  MatrixMultiply : Product  Multiplication=Matrix(*)
  Mux : Mux  Inputs=3
  Mux1 : Mux  Inputs=3
  Sqrt : Sqrt  SaturateOnIntegerOverflow=on
  Sum1 : Sum  Inputs=|++-
  Sum2 : Sum  Inputs=|+++
  l : Outport
  wires:
  Demux/1 -> Mux/1
  Demux/2 -> Mux/2
  Demux/3 -> Mux/3
  Demux/4 -> Mux1/1
  Demux/5 -> Mux1/2
  Demux/6 -> Mux1/3
  Coordinates(2)/1 -> Demux/1
  Mux1/1 -> MatrixMultiply/2  "p1"
  Mux/1 -> Sum1/3  "b1"
  pRb/1 -> MatrixMultiply/1
  MatrixMultiply/1 -> Sum1/2
  Translatie/1 -> Sum1/1
  Sum2/1 -> Sqrt/1
  Sum1/1 -> Demux1/1
  Math Function11/1 -> Sum2/1
  Math Function3/1 -> Sum2/3
  Sqrt/1 -> l/1
  Demux1/1 -> Math Function11/1
  Demux1/2 -> Math Function2/1
  Math Function2/1 -> Sum2/2
  Demux1/3 -> Math Function3/1

== system SCAUN_NOBIL/Leg length calculator/l3 calc ==
  Translatie : Inport
  pRb : Inport  Port=2
  Coordinates(3) : Inport  Port=3
  Demux : Demux  Outputs=6
  Demux1 : Demux  Outputs=3
  Math Function11 : Math  Operator=magnitude^2  SaturateOnIntegerOverflow=on
  Math Function2 : Math  Operator=magnitude^2  SaturateOnIntegerOverflow=on
  Math Function3 : Math  Operator=magnitude^2  SaturateOnIntegerOverflow=on
  MatrixMultiply : Product  Multiplication=Matrix(*)
  Mux : Mux  Inputs=3
  Mux1 : Mux  Inputs=3
  Sqrt : Sqrt  SaturateOnIntegerOverflow=on
  Sum1 : Sum  Inputs=|++-
  Sum2 : Sum  Inputs=|+++
  l1 : Outport
  wires:
  Demux/1 -> Mux/1
  Demux/2 -> Mux/2
  Demux/3 -> Mux/3
  Demux/4 -> Mux1/1
  Demux/5 -> Mux1/2
  Demux/6 -> Mux1/3
  Coordinates(3)/1 -> Demux/1
  Mux1/1 -> MatrixMultiply/2  "p1"
  Mux/1 -> Sum1/3  "b1"
  pRb/1 -> MatrixMultiply/1
  MatrixMultiply/1 -> Sum1/2
  Translatie/1 -> Sum1/1
  Math Function2/1 -> Sum2/2
  Demux1/3 -> Math Function3/1
  Math Function11/1 -> Sum2/1
  Demux1/1 -> Math Function11/1
  Sum2/1 -> Sqrt/1
  Sqrt/1 -> l1/1
  Sum1/1 -> Demux1/1
  Math Function3/1 -> Sum2/3
  Demux1/2 -> Math Function2/1

== system SCAUN_NOBIL/Leg length calculator/l4 calc ==
  Translatie : Inport
  pRb : Inport  Port=2
  Coordinates(4) : Inport  Port=3
  Demux : Demux  Outputs=6
  Demux1 : Demux  Outputs=3
  Math Function11 : Math  Operator=magnitude^2  SaturateOnIntegerOverflow=on
  Math Function2 : Math  Operator=magnitude^2  SaturateOnIntegerOverflow=on
  Math Function3 : Math  Operator=magnitude^2  SaturateOnIntegerOverflow=on
  MatrixMultiply : Product  Multiplication=Matrix(*)
  Mux : Mux  Inputs=3
  Mux1 : Mux  Inputs=3
  Sqrt : Sqrt  SaturateOnIntegerOverflow=on
  Sum1 : Sum  Inputs=|++-
  Sum2 : Sum  Inputs=|+++
  l : Outport
  wires:
  Demux/1 -> Mux/1
  Demux/2 -> Mux/2
  Demux/3 -> Mux/3
  Demux/4 -> Mux1/1
  Demux/5 -> Mux1/2
  Demux/6 -> Mux1/3
  Coordinates(4)/1 -> Demux/1
  Mux1/1 -> MatrixMultiply/2  "p1"
  Mux/1 -> Sum1/3  "b1"
  pRb/1 -> MatrixMultiply/1
  MatrixMultiply/1 -> Sum1/2
  Translatie/1 -> Sum1/1
  Math Function2/1 -> Sum2/2
  Demux1/3 -> Math Function3/1
  Math Function11/1 -> Sum2/1
  Demux1/1 -> Math Function11/1
  Sum2/1 -> Sqrt/1
  Sqrt/1 -> l/1
  Sum1/1 -> Demux1/1
  Math Function3/1 -> Sum2/3
  Demux1/2 -> Math Function2/1

== system SCAUN_NOBIL/Leg length calculator/l5 calc ==
  Translatie : Inport
  pRb : Inport  Port=2
  Coordinates(5) : Inport  Port=3
  Demux : Demux  Outputs=6
  Demux1 : Demux  Outputs=3
  Math Function11 : Math  Operator=magnitude^2  SaturateOnIntegerOverflow=on
  Math Function2 : Math  Operator=magnitude^2  SaturateOnIntegerOverflow=on
  Math Function3 : Math  Operator=magnitude^2  SaturateOnIntegerOverflow=on
  MatrixMultiply : Product  Multiplication=Matrix(*)
  Mux : Mux  Inputs=3
  Mux1 : Mux  Inputs=3
  Sqrt : Sqrt  SaturateOnIntegerOverflow=on
  Sum1 : Sum  Inputs=|++-
  Sum2 : Sum  Inputs=|+++
  l : Outport
  wires:
  Demux/1 -> Mux/1
  Demux/2 -> Mux/2
  Demux/3 -> Mux/3
  Demux/4 -> Mux1/1
  Demux/5 -> Mux1/2
  Demux/6 -> Mux1/3
  Coordinates(5)/1 -> Demux/1
  Mux1/1 -> MatrixMultiply/2  "p1"
  Mux/1 -> Sum1/3  "b1"
  pRb/1 -> MatrixMultiply/1
  MatrixMultiply/1 -> Sum1/2
  Translatie/1 -> Sum1/1
  Math Function2/1 -> Sum2/2
  Demux1/3 -> Math Function3/1
  Math Function11/1 -> Sum2/1
  Demux1/1 -> Math Function11/1
  Sum2/1 -> Sqrt/1
  Sum1/1 -> Demux1/1
  Math Function3/1 -> Sum2/3
  Demux1/2 -> Math Function2/1
  Sqrt/1 -> l/1

== system SCAUN_NOBIL/Leg length calculator/l6 calc ==
  Translatie : Inport
  pRb : Inport  Port=2
  Coordinates(6) : Inport  Port=3
  Demux : Demux  Outputs=6
  Demux1 : Demux  Outputs=3
  Math Function11 : Math  Operator=magnitude^2  SaturateOnIntegerOverflow=on
  Math Function2 : Math  Operator=magnitude^2  SaturateOnIntegerOverflow=on
  Math Function3 : Math  Operator=magnitude^2  SaturateOnIntegerOverflow=on
  MatrixMultiply : Product  Multiplication=Matrix(*)
  Mux : Mux  Inputs=3
  Mux1 : Mux  Inputs=3
  Sqrt : Sqrt  SaturateOnIntegerOverflow=on
  Sum1 : Sum  Inputs=|++-
  Sum2 : Sum  Inputs=|+++
  l : Outport
  wires:
  Demux/1 -> Mux/1
  Demux/2 -> Mux/2
  Demux/3 -> Mux/3
  Demux/4 -> Mux1/1
  Demux/5 -> Mux1/2
  Demux/6 -> Mux1/3
  Coordinates(6)/1 -> Demux/1
  Mux1/1 -> MatrixMultiply/2  "p1"
  Mux/1 -> Sum1/3  "b1"
  pRb/1 -> MatrixMultiply/1
  MatrixMultiply/1 -> Sum1/2
  Translatie/1 -> Sum1/1
  Math Function2/1 -> Sum2/2
  Demux1/3 -> Math Function3/1
  Math Function11/1 -> Sum2/1
  Demux1/1 -> Math Function11/1
  Sum2/1 -> Sqrt/1
  Sum1/1 -> Demux1/1
  Math Function3/1 -> Sum2/3
  Demux1/2 -> Math Function2/1
  Sqrt/1 -> l/1
